simulink model "ACC_TESTE_2026"  (R2025b)
settings: Solver=VariableStepAuto  StartTime=0.0  StopTime=10.0  RelTol=1e-3
values from neighbouring files (symbols this model uses):
  D0 = 150    [INIT_ACC_2026.m]
  Vf0 = 18    [INIT_ACC_2026.m]
settings Model: Creator=ADM  LastModifiedBy=Dell
settings DataIOCC: ReturnWorkspaceOutputs=off

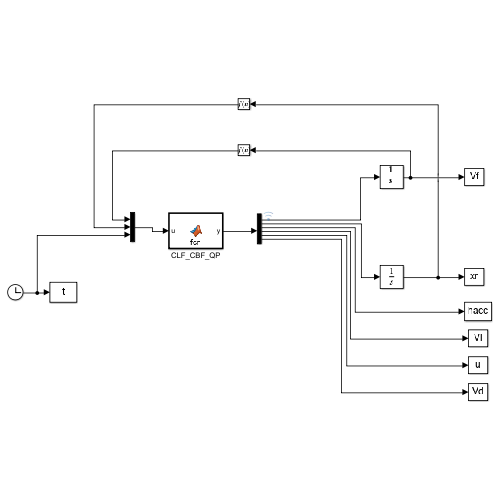
[thumbnail: Simulink's stored preview of the top-level diagram]
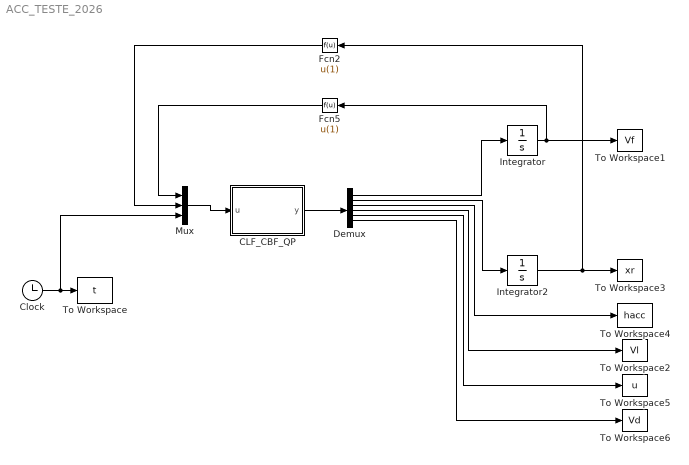
== system ACC_TESTE_2026 ==
  CLF_CBF_QP : MATLAB Function  TreatAsAtomicUnit=on
  Clock : Clock
  Demux : Demux  Outputs=6
  Fcn2 : Fcn  Expr=u(1)
  Fcn5 : Fcn  Expr=u(1)
  Integrator : Integrator  InitialCondition=Vf0
  Integrator2 : Integrator  InitialCondition=D0
  Mux : Mux  Inputs=3
  To Workspace : ToWorkspace  VariableName=t  SampleTime=-1
  To Workspace1 : ToWorkspace  VariableName=Vf  SampleTime=-1
  To Workspace2 : ToWorkspace  VariableName=Vl  SampleTime=-1
  To Workspace3 : ToWorkspace  VariableName=xr  SampleTime=-1
  To Workspace4 : ToWorkspace  VariableName=hacc  SampleTime=-1
  To Workspace5 : ToWorkspace  VariableName=u  SampleTime=-1
  To Workspace6 : ToWorkspace  VariableName=Vd  SampleTime=-1
  wires:
  CLF_CBF_QP/1(y) -> Demux/1
  Clock/1 -> Mux/3, To Workspace/1
  Integrator2/1 -> To Workspace3/1, Fcn2/1
  Demux/1 -> Integrator/1
  Demux/4 -> To Workspace2/1
  Fcn2/1 -> Mux/2
  Demux/2 -> Integrator2/1
  Mux/1 -> CLF_CBF_QP/1(u)
  Integrator/1 -> To Workspace1/1, Fcn5/1
  Demux/3 -> To Workspace4/1
  Fcn5/1 -> Mux/1
  Demux/5 -> To Workspace5/1
  Demux/6 -> To Workspace6/1

== matlab function ACC_TESTE_2026/CLF_CBF_QP ==
  data: u input; y output
function y = fcn(u)
% ============================================================
% ACC — CLF-CBF-QP completo (Ames, Grizzle & Tabuada, 2014)
% "Case I": CLF (velocidade) + CBF (distância segura), SEM
% restrições de força/conforto (h_F não implementada aqui).
% Convenção de unidades: u é FORÇA (N)  =>  m*dVf/dt = Fw - Fr
% ============================================================

% Estados
Vf = u(1);
xr = u(2);
% Tempo
t  = u(3);

% --- Parâmetros do veículo (Tabela I, Ames et al. 2014) ---
m  = 1650;
f0 = 0.1;
f1 = 5;
f2 = 0.25;

% --- Perfil do veículo líder (mantido customizado, ver simulacao.md) ---
if(t <= 10)
    Vl = 10;
elseif(t>10 && t<=20)
    Vl = -2+1.2*t;
elseif(t>20 && t<=30)
    Vl = 22;
elseif(t>30 && t<=40)
    Vl = 7+0.5*t;
elseif(t>40 && t<=50)
    Vl = 27;
elseif(t>50 && t<=60)
    Vl = 77-t;
else
    Vl = 17;
end

% --- Força de arrasto aerodinâmico ---
Fr = f0 + f1*Vf + f2*Vf*Vf;

% --- Sistema no espaço de estados: x=[Vf;xr], u = Fw (N) ---
f = [-Fr/m; Vl-Vf];
g = [1/m; 0];

% --- Parâmetros de projeto (Tabela I, Ames et al. 2014) ---
Vd  = 22;      % mantido em 22 (escolha do autor; artigo usa 24)
psc = 10;    % peso da folga delta — validado (ver simulacao.md, Seção 1.2)
c   = 10;      % taxa de convergência da CLF (≡ ε no artigo)
lambda = 1;    % agressividade da CBF na fronteira (≡ γ no artigo)
Td  = 1.8;     % time headway (≡ τd no artigo)

% --- CLF: rastreamento da velocidade de cruzeiro ---
Vacc = (Vf-Vd)^2;
LfVacc = (Fr*(2*Vd - 2*Vf))/m;
LgVacc = (2*Vf - 2*Vd)/m;

% --- CBF: distância segura (time headway) ---
hacc = xr - Td*Vf;
Lfhacc = Vl - Vf + (Fr*Td)/m;
Lghacc = -Td/m;

% --- Custo do QP (min-norm em torno de Fr, escala de força) ---
Hacc = 2*[1/(m*m) 0; 0 psc];
Facc = -2*[Fr/(m*m); 0];

% --- Restrições: CLF (suave, com folga) + CBF (rígida) ---
A = [LgVacc -1; -Lghacc 0];
b = [-LfVacc-c*Vacc; Lfhacc+lambda*(hacc)];

% --- Resolve o QP ---
ucont = [0;0];
coder.extrinsic('QPhild');
ucont = QPhild(Hacc,Facc,A,b);

% --- Aplica o controle ---
xponto = f + g.*ucont(1,1);
y = [xponto(1,1); xponto(2,1); hacc; Vl; ucont(1,1); Vd];
